simulink model "sampleModel1693"  (R2023a)
settings: Solver=VariableStepAuto  StartTime=0.0  StopTime=10.0  RelTol=1e-3
libraries: hdlsllib x8, simulink x1
settings Model: Creator=user1  LastModifiedBy=user1

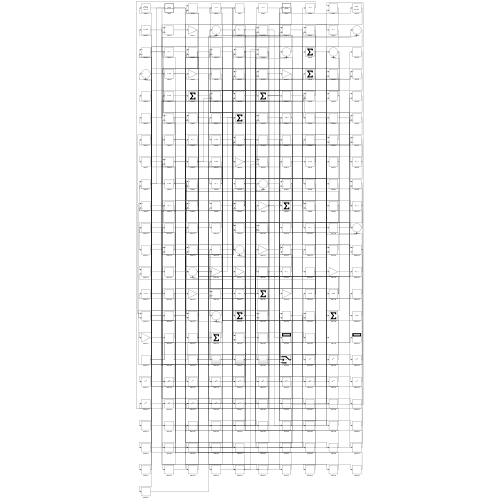
[thumbnail: Simulink's stored preview of the top-level diagram]
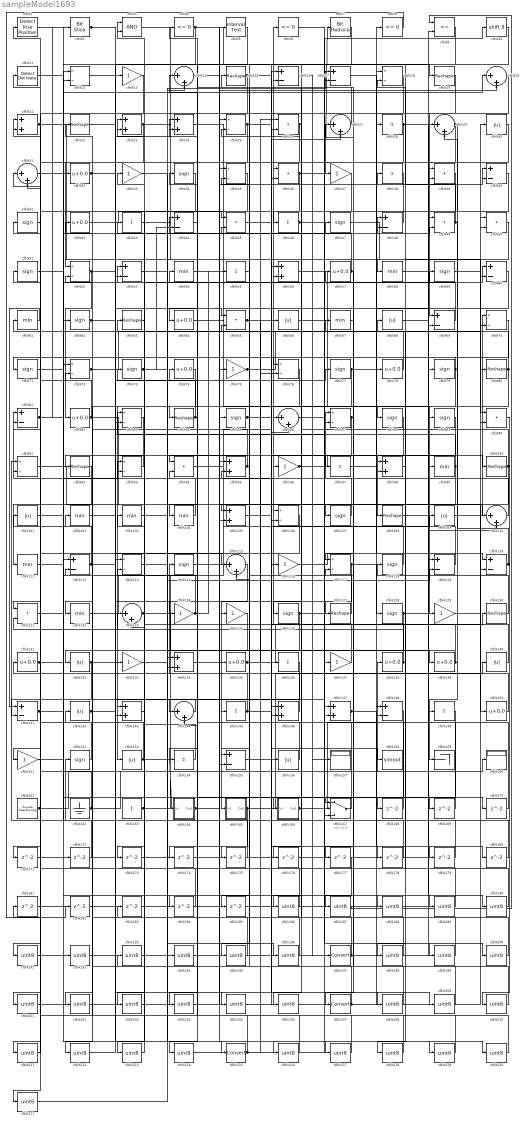
== system sampleModel1693 ==
  cfblk1 : hdlsllib/Logic and Bit Operations/Detect Rise Positive  vinit=0  OutDataTypeStr=boolean
  cfblk10 : ArithShift  BitShiftNumber=8
  cfblk{15,19,22,63,80,84,92,100,108,127,130} (11 alike) : Reshape
  cfblk{30,66,68,101,109,132,140,142,153,156} (10 alike) : Abs  SaturateOnIntegerOverflow=off
  cfblk{54,58,61,67,99,102..104,111,122} (10 alike) : MinMax
  cfblk{21,23..24,56,95,98,105,134,143,146..147} (11 alike) : Sum
  cfblk{12,18,25,35,52,70,72,76,83,87,91,93,106,113,117} (15 alike) : Product  Inputs=*/  RndMeth=Zero  SaturateOnIntegerOverflow=on
  cfblk{34,41,47,51,59,62,71,73,77,79,85,88..89,107,114,118,126,128,152} (19 alike) : Signum
  cfblk11 : simulink/Logic and Bit Operations/Detect Decrease  vinit=0.0  OutDataTypeStr=boolean
      settings: LibrarySourceBlock=|
      | hdlsllib/Logic and Bit
      | Operations/Detect
      | Decrease
  cfblk{14,20,27,29,31,86,110,115,123,144} (10 alike) : Sum  Inputs=|++
  cfblk{16..17,40,44,48,53,60,69,81,112,119..120,141,148,155} (15 alike) : Sum  Inputs=+-
  cfblk{13,33,37,75,96,116,124..125,129,133,137,151} (12 alike) : Gain
  cfblk{26,36,39,45,49..50,65,90,94,121} (10 alike) : DotProduct  OutDataTypeStr=Inherit: Inherit via internal rule
  cfblk{32,42,57,64,74,78,82,131,135,138..139,150} (12 alike) : Bias  Bias=0.0  SaturateOnIntegerOverflow=off
  cfblk{28,38,43,46,55,97,136,145,149,154} (10 alike) : Sum  Inputs=+
  cfblk157 : Display
  cfblk158 : ToWorkspace  VariableName=simout  SaveFormat=Timeseries  SampleTime=-1
  cfblk159 : Terminator
  cfblk160 : Display
  cfblk161 : hdlsllib/Sources/Counter Free-Running  NumBits=16  tsamp=-1
  cfblk162 : Ground
  cfblk163 : Constant  SampleTime=-1
  cfblk164 : Subsystem
      settings: LibrarySourceBlock=|
      | hdlsllib/Ports &
      | Subsystems/Subsystem
  cfblk165 : Subsystem
      settings: LibrarySourceBlock=|
      | hdlsllib/Ports &
      | Subsystems/Subsystem
  cfblk166 : Subsystem
      settings: LibrarySourceBlock=|
      | hdlsllib/Ports &
      | Subsystems/Subsystem
  cfblk167 : Switch  SaturateOnIntegerOverflow=off  InputSameDT=off
  cfblk{168..185} (18 alike) : Delay  SampleTime=1
  cfblk{186..196,198..206,208..214,216..221} (33 alike) : DataTypeConversion  OutDataTypeStr=uint8  SaturateOnIntegerOverflow=off  RndMeth=Floor
  cfblk197 : DataTypeConversion  SaturateOnIntegerOverflow=off  RndMeth=Floor
  cfblk2 : hdlsllib/Logic and Bit Operations/Bit Slice  lidx=7  ridx=0
  cfblk207 : DataTypeConversion  SaturateOnIntegerOverflow=off  RndMeth=Floor
  cfblk215 : DataTypeConversion  SaturateOnIntegerOverflow=off  RndMeth=Floor
  cfblk3 : Logic  AllPortsSameDT=off  OutDataTypeStr=boolean
  cfblk4 : hdlsllib/Logic and Bit Operations/Compare To Zero  relop=<=  OutDataTypeStr=boolean
  cfblk5 : hdlsllib/Logic and Bit Operations/Interval Test  IntervalClosedRight=on  uplimit=0.5  IntervalClosedLeft=on  lowlimit=-0.5  OutDataTypeStr=boolean
  cfblk6 : hdlsllib/Logic and Bit Operations/Compare To Zero  relop=<=  OutDataTypeStr=boolean
  cfblk7 : hdlsllib/Logic and Bit Operations/Bit Reduce  mode=AND
  cfblk8 : hdlsllib/Logic and Bit Operations/Compare To Zero  relop=<=  OutDataTypeStr=boolean
  cfblk9 : RelationalOperator  Operator=<=  OutDataTypeStr=boolean  InputSameDT=off
  wires:
  cfblk156/1 -> cfblk74/1
  cfblk19/1 -> cfblk69/1
  cfblk139/1 -> cfblk6/1, cfblk132/1, cfblk24/2
  cfblk91/1 -> cfblk107/1
  cfblk128/1 -> cfblk190/1, cfblk206/1
  cfblk127/1 -> cfblk63/1
  cfblk3/1 -> cfblk58/1
  cfblk54/1 -> cfblk69/2
  cfblk107/1 -> cfblk81/1
  cfblk146/1 -> cfblk114/1
  cfblk24/1 -> cfblk129/1
  cfblk88/1 -> cfblk108/1
  cfblk118/1 -> cfblk106/1
  cfblk28/1 -> cfblk52/1, cfblk110/2
  cfblk94/1 -> cfblk98/1
  cfblk87/1 -> cfblk117/1, cfblk176/1
  cfblk93/1 -> cfblk92/1
  cfblk115/1 -> cfblk165/1(In1)
  cfblk5/1 -> cfblk84/1
  cfblk18/1 -> cfblk145/1
  cfblk84/1 -> cfblk54/1, cfblk23/2
  cfblk40/1 -> cfblk64/1
  cfblk57/1 -> cfblk36/1, cfblk97/1
  cfblk17/1 -> cfblk78/1
  cfblk74/1 -> cfblk153/1
  cfblk114/1 -> cfblk96/1
  cfblk69/1 -> cfblk3/1
  cfblk16/1 -> cfblk197/1
  cfblk79/1 -> cfblk126/1, cfblk76/1
  cfblk53/1 -> cfblk139/1
  cfblk73/1 -> cfblk44/2, cfblk196/1
  cfblk145/1 -> cfblk21/1, cfblk27/2
  cfblk36/1 -> cfblk7/1, cfblk105/2
  cfblk123/1 -> cfblk167/3, cfblk188/1
  cfblk134/1 -> cfblk35/1
  cfblk163/1 -> cfblk109/1, cfblk119/2
  cfblk90/1 -> cfblk152/1
  cfblk65/1 -> cfblk147/2, cfblk136/1
  cfblk92/1 -> cfblk111/1
  cfblk15/1 -> cfblk151/1, cfblk178/1
  cfblk49/1 -> cfblk159/1, cfblk18/2
  cfblk27/1 -> cfblk4/1
  cfblk165/1(Out1) -> cfblk140/1, cfblk76/2, cfblk214/1
  cfblk109/1 -> cfblk70/1
  cfblk56/1 -> cfblk89/1
  cfblk60/1 -> cfblk98/2
  cfblk68/1 -> cfblk149/1
  cfblk38/1 -> cfblk144/1
  cfblk76/1 -> cfblk104/1
  cfblk103/1 -> cfblk134/1
  cfblk50/1 -> cfblk88/1
  cfblk21/1 -> cfblk156/1, cfblk20/1
  cfblk12/1 -> cfblk19/1
  cfblk126/1 -> cfblk49/2, cfblk185/1
  cfblk29/1 -> cfblk49/1, cfblk36/2
  cfblk153/1 -> cfblk164/1(In1), cfblk41/1
  cfblk25/1 -> cfblk83/2, cfblk155/1, cfblk208/1
  cfblk64/1 -> cfblk119/1
  cfblk23/1 -> cfblk80/1, cfblk143/2, cfblk32/1
  cfblk143/1 -> cfblk3/2
  cfblk116/1 -> cfblk120/1
  cfblk100/1 -> cfblk43/1, cfblk198/1
  cfblk32/1 -> cfblk65/1, cfblk115/1
  cfblk85/1 -> cfblk59/1, cfblk40/1
  cfblk22/1 -> cfblk215/1
  cfblk140/1 -> cfblk61/1
  cfblk129/1 -> cfblk70/2
  cfblk155/1 -> cfblk116/1
  cfblk162/1 -> cfblk138/1, cfblk31/2
  cfblk111/1 -> cfblk53/1
  cfblk48/1 -> cfblk46/1
  cfblk144/1 -> cfblk143/1
  cfblk133/1 -> cfblk17/1
  cfblk97/1 -> cfblk28/1
  cfblk135/1 -> cfblk30/1, cfblk130/1
  cfblk138/1 -> cfblk23/1, cfblk121/2
  cfblk52/1 -> cfblk82/1, cfblk205/1
  cfblk80/1 -> cfblk34/1, cfblk203/1
  cfblk95/1 -> cfblk94/1, cfblk72/2
  cfblk31/1 -> cfblk75/1
  cfblk110/1 -> cfblk87/1
  cfblk59/1 -> cfblk90/1
  cfblk167/1 -> cfblk15/1
  cfblk104/1 -> cfblk31/1
  cfblk122/1 -> cfblk48/1
  cfblk45/1 -> cfblk158/1
  cfblk154/1 -> cfblk103/1
  cfblk120/1 -> cfblk29/2, cfblk210/1
  cfblk124/1 -> cfblk112/2, cfblk55/1
  cfblk2/1 -> cfblk133/1, cfblk146/2
  cfblk26/1 -> cfblk71/1, cfblk25/2
  cfblk51/1 -> cfblk12/1
  cfblk81/1 -> cfblk47/1, cfblk2/1
  cfblk89/1 -> cfblk106/2
  cfblk131/1 -> cfblk62/1, cfblk184/1
  cfblk63/1 -> cfblk123/2
  cfblk70/1 -> cfblk121/1
  cfblk42/1 -> cfblk45/1
  cfblk166/1(Out1) -> cfblk8/1, cfblk160/1
  cfblk20/1 -> cfblk154/1
  cfblk67/1 -> cfblk207/1
  cfblk4/1 -> cfblk146/1, cfblk20/2, cfblk12/2
  cfblk82/1 -> cfblk150/1, cfblk137/1, cfblk51/1
  cfblk152/1 -> cfblk101/1
  cfblk130/1 -> cfblk118/1
  cfblk72/1 -> cfblk50/1, cfblk124/1
  cfblk43/1 -> cfblk135/1
  cfblk161/1 -> cfblk134/2, cfblk60/2
  cfblk46/1 -> cfblk10/1, cfblk40/2, cfblk180/1
  cfblk112/1 -> cfblk91/2, cfblk24/1
  cfblk62/1 -> cfblk127/1, cfblk167/1
  cfblk151/1 -> cfblk93/1
  cfblk96/1 -> cfblk100/1, cfblk157/1
  cfblk61/1 -> cfblk141/1
  cfblk132/1 -> cfblk56/2, cfblk171/1
  cfblk44/1 -> cfblk144/2
  cfblk75/1 -> cfblk50/2, cfblk35/2
  cfblk117/1 -> cfblk128/1, cfblk167/2
  cfblk150/1 -> cfblk44/1
  cfblk147/1 -> cfblk57/1, cfblk179/1
  cfblk119/1 -> cfblk27/1
  cfblk136/1 -> cfblk141/2
  cfblk99/1 -> cfblk83/1, cfblk115/2, cfblk155/2
  cfblk108/1 -> cfblk60/1
  cfblk137/1 -> cfblk73/1
  cfblk164/1(Out1) -> cfblk5/1, cfblk38/1
  cfblk78/1 -> cfblk65/2
  cfblk105/1 -> cfblk110/1
  cfblk47/1 -> cfblk99/1
  cfblk142/1 -> cfblk77/1, cfblk87/2
  cfblk55/1 -> cfblk105/1
  cfblk141/1 -> cfblk48/2, cfblk166/1(In1)
  cfblk77/1 -> cfblk120/2, cfblk122/1
  cfblk98/1 -> cfblk168/1
  cfblk168/1 -> cfblk94/2
  cfblk86/1 -> cfblk169/1
  cfblk169/1 -> cfblk123/1
  cfblk58/1 -> cfblk170/1
  cfblk170/1 -> cfblk112/1
  cfblk171/1 -> cfblk53/2
  cfblk121/1 -> cfblk172/1
  cfblk172/1 -> cfblk72/1
  cfblk34/1 -> cfblk173/1
  cfblk173/1 -> cfblk25/1
  cfblk35/1 -> cfblk174/1
  cfblk174/1 -> cfblk29/1
  cfblk7/1 -> cfblk175/1
  cfblk175/1 -> cfblk21/2
  cfblk176/1 -> cfblk147/1
  cfblk149/1 -> cfblk177/1
  cfblk178/1 -> cfblk117/2
  cfblk179/1 -> cfblk81/2
  cfblk180/1 -> cfblk91/1
  cfblk181/1 -> cfblk95/1
  cfblk8/1 -> cfblk182/1
  cfblk182/1 -> cfblk18/1
  cfblk183/1 -> cfblk26/2
  cfblk184/1 -> cfblk1/1
  cfblk185/1 -> cfblk79/1
  cfblk9/1 -> cfblk186/1
  cfblk186/1 -> cfblk142/1
  cfblk177/1 -> cfblk187/1
  cfblk187/1 -> cfblk9/1
  cfblk188/1 -> cfblk9/2
  cfblk11/1 -> cfblk189/1
  cfblk189/1 -> cfblk68/1
  cfblk190/1 -> cfblk11/1
  cfblk39/1 -> cfblk191/1
  cfblk191/1 -> cfblk56/1
  cfblk101/1 -> cfblk192/1
  cfblk192/1 -> cfblk39/1
  cfblk193/1 -> cfblk39/2
  cfblk113/1 -> cfblk194/1
  cfblk194/1 -> cfblk86/2
  cfblk30/1 -> cfblk195/1
  cfblk195/1 -> cfblk113/1
  cfblk196/1 -> cfblk113/2
  cfblk197/1 -> cfblk52/2, cfblk86/1
  cfblk198/1 -> cfblk16/1
  cfblk6/1 -> cfblk199/1
  cfblk199/1 -> cfblk16/2
  cfblk66/1 -> cfblk200/1
  cfblk200/1 -> cfblk17/2
  cfblk41/1 -> cfblk201/1
  cfblk201/1 -> cfblk66/1
  cfblk125/1 -> cfblk202/1
  cfblk202/1 -> cfblk85/1
  cfblk203/1 -> cfblk125/1
  cfblk148/1 -> cfblk204/1
  cfblk204/1 -> cfblk90/2
  cfblk205/1 -> cfblk148/1
  cfblk206/1 -> cfblk148/2
  cfblk207/1 -> cfblk45/2, cfblk95/2
  cfblk208/1 -> cfblk67/1
  cfblk102/1 -> cfblk209/1
  cfblk209/1 -> cfblk93/2
  cfblk210/1 -> cfblk102/1
  cfblk13/1 -> cfblk211/1
  cfblk211/1 -> cfblk131/1
  cfblk83/1 -> cfblk212/1
  cfblk212/1 -> cfblk13/1
  cfblk37/1 -> cfblk213/1
  cfblk213/1 -> cfblk183/1
  cfblk214/1 -> cfblk37/1
  cfblk215/1 -> cfblk193/1, cfblk26/1
  cfblk1/1 -> cfblk216/1
  cfblk216/1 -> cfblk22/1
  cfblk33/1 -> cfblk217/1
  cfblk217/1 -> cfblk181/1
  cfblk10/1 -> cfblk218/1
  cfblk218/1 -> cfblk33/1
  cfblk14/1 -> cfblk219/1
  cfblk219/1 -> cfblk42/1
  cfblk71/1 -> cfblk220/1
  cfblk220/1 -> cfblk14/1
  cfblk106/1 -> cfblk221/1
  cfblk221/1 -> cfblk14/2

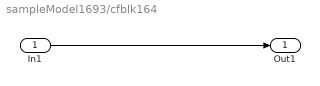
== system sampleModel1693/cfblk164 ==
  In1 : Inport
  Out1 : Outport
  wires:
  In1/1 -> Out1/1

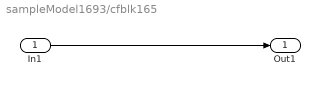
== system sampleModel1693/cfblk165 ==
  In1 : Inport
  Out1 : Outport
  wires:
  In1/1 -> Out1/1

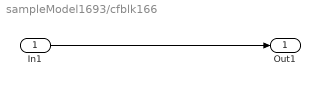
== system sampleModel1693/cfblk166 ==
  In1 : Inport
  Out1 : Outport
  wires:
  In1/1 -> Out1/1
